simulink model "opc_simple_teste"  (R2013a)
settings: Solver=ode45  StartTime=0.0  StopTime=Inf  RelTol=1e-3
undefined symbols (not defined in the file): Bomba1, Bomba2, Opc_Teste, Tanq1, Tanq2, Tanq3, Tanq4
libraries: opclib x3
settings Model: Creator=Administrator  LastModifiedBy=Administrator

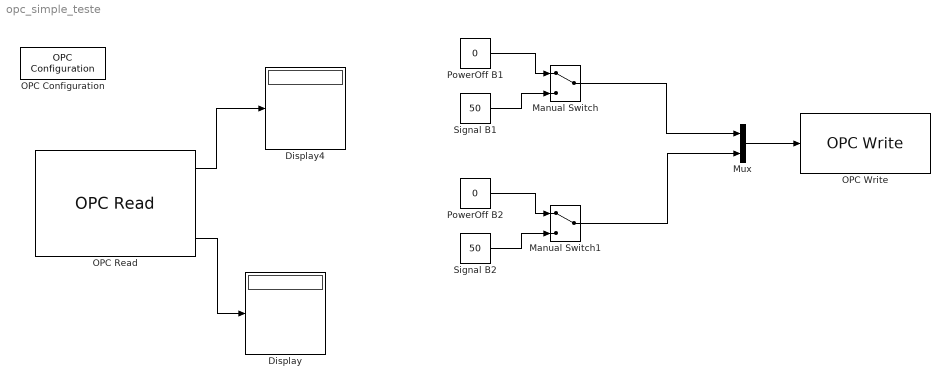
== system opc_simple_teste ==
  Display : Display
  Display4 : Display
  Manual Switch : ManualSwitch
  Manual Switch1 : ManualSwitch
  Mux : Mux  Inputs=2
  OPC Configuration : opclib/OPC Configuration  opcServers=localhost/RSLinx OPC Server/10  errMissingItems=Error  errReadWrite=Warn  errShutdown=Error  errRTViolation=Warn  rtEnable=on  speedup=1  showLatency=off  beingUsed=on
  OPC Read : opclib/OPC Read  serverHost=localhost  serverID=RSLinx OPC Server  itemIDs=[Opc_Teste]Tanq4, [Opc_Teste]Tanq3, [Opc_Teste]Tanq2, [Opc_Teste]Tanq1  readMode=Synchronous (cache)  dataType=double  updateRate=0.5  showQual=on  showTS=on  tsMode=Seconds since start
  OPC Write : opclib/OPC Write  serverHost=localhost  serverID=RSLinx OPC Server  itemIDs=[Opc_Teste]Bomba1, [Opc_Teste]Bomba2  writeMode=Synchronous  updateRate=0
  PowerOff B1 : Constant  Value=0
  PowerOff B2 : Constant  Value=0
  Signal B1 : Constant  Value=50
  Signal B2 : Constant  Value=50
  wires:
  OPC Read/3 -> Display/1
  OPC Read/1 -> Display4/1
  PowerOff B1/1 -> Manual Switch/1
  Signal B1/1 -> Manual Switch/2
  PowerOff B2/1 -> Manual Switch1/1
  Signal B2/1 -> Manual Switch1/2
  Manual Switch/1 -> Mux/1
  Manual Switch1/1 -> Mux/2
  Mux/1 -> OPC Write/1
